simulink model "idiot_block"  (R2022b)
settings: Solver=VariableStepAuto  StartTime=0.0  StopTime=10.0  RelTol=1e-3
settings Model: Creator=yeyi5  LastModifiedBy=yeyi5

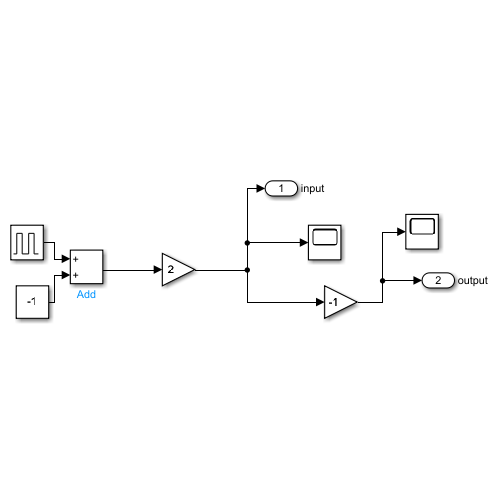
[thumbnail: Simulink's stored preview of the top-level diagram]
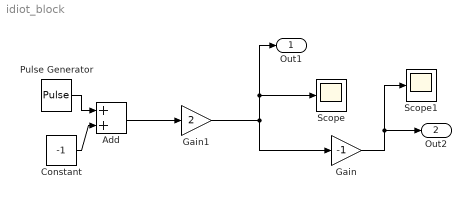
== system idiot_block ==
  Add : Sum
  Constant : Constant  Value=-1
  Gain : Gain  Gain=-1
  Gain1 : Gain  Gain=2
  Pulse Generator : DiscretePulseGenerator  PulseType=Time based  Amplitude=2  Period=1/0.5  PulseWidth=50
  Scope : Scope
  Scope1 : Scope
  Out1 : Outport  SignalName=input
  Out2 : Outport  Port=2  SignalName=output
  wires:
  Gain/1 -> Out2/1, Scope1/1
  Pulse Generator/1 -> Add/1
  Constant/1 -> Add/2
  Add/1 -> Gain1/1
  Gain1/1 -> Scope/1, Out1/1, Gain/1
